simulink model "Feeder_1"  (Simulink 8.8)
settings: Solver=ode4  StartTime=0.0  StopTime=inf  FixedStep=Ts  RelTol=1e-3  EnableMultiTasking=on
PreLoadFcn:
  | Ts=125e-6;Core_Num = 0; np=1; nq=1; Vmin=.9;
PostLoadFcn:
  | Ts=125e-6;Core_Num = 0; np=1; nq=1; Vmin=.9;
InitFcn:
  | Ts=125e-6;Core_Num = 0; np=1; nq=1; Vmin=.9;
undefined symbols (not defined in the file or in its folder): another_event_name, DiscIntNeverNeededParam, I, j, Left, my_event_name, Right, type, V, X
libraries: powerlib x316, powerlib_meascontrol x227, simulink_extras x78, simulink x25, rtio_generic_c37_118 x22, ssn_lib x9, rtlab x6, powerlib_extras x3, artemis x1, rtio_opalrt_ml605ex1 x1, rtio_spectracom x1, rtio_generic_ethernet x1
(part 4 of 14)

== system Feeder_1/SM_NG/Single-Phase Dynamic Load36 ==
  PQ : Inport
  Controlled Current Source : powerlib/Electrical Sources/Controlled Current Source  Initialize=on  Source_Type=AC  Amplitude=0  Phase=0  Frequency=0  Measurements=None
  Ground52 : powerlib/Elements/Ground  LConnTagsString=a
  Voltage Measurement1 : powerlib/Measurements/Voltage Measurement  PhasorSimulation=off  OutputType=Complex  PSBequivalent=0
  model : Subsystem
  a : PMIOPort  Tag=PMCPort  Port=1  Side=Right
  wires:
  PQ/1 -> model/2(PQ)
  Voltage Measurement1/1 -> model/1(v)
  model/1(i) -> Controlled Current Source/1
  connections:
  Voltage Measurement1/LConn1 -- a/RConn1 -- Controlled Current Source/RConn1
  Voltage Measurement1/LConn2 -- Ground52/LConn1 -- Controlled Current Source/LConn1

== system Feeder_1/SM_NG/Single-Phase Dynamic Load37 ==
  PQ : Inport
  Controlled Current Source : powerlib/Electrical Sources/Controlled Current Source  Initialize=on  Source_Type=AC  Amplitude=0  Phase=0  Frequency=0  Measurements=None
  Ground52 : powerlib/Elements/Ground  LConnTagsString=a
  Voltage Measurement1 : powerlib/Measurements/Voltage Measurement  PhasorSimulation=off  OutputType=Complex  PSBequivalent=0
  model : Subsystem
  a : PMIOPort  Tag=PMCPort  Port=1  Side=Right
  wires:
  PQ/1 -> model/2(PQ)
  Voltage Measurement1/1 -> model/1(v)
  model/1(i) -> Controlled Current Source/1
  connections:
  Voltage Measurement1/LConn1 -- a/RConn1 -- Controlled Current Source/RConn1
  Ground52/LConn1 -- Voltage Measurement1/LConn2 -- Controlled Current Source/LConn1

== system Feeder_1/SM_NG/Single-Phase Dynamic Load38 ==
  PQ : Inport
  Controlled Current Source : powerlib/Electrical Sources/Controlled Current Source  Initialize=on  Source_Type=AC  Amplitude=0  Phase=0  Frequency=0  Measurements=None
  Ground52 : powerlib/Elements/Ground  LConnTagsString=a
  Voltage Measurement1 : powerlib/Measurements/Voltage Measurement  PhasorSimulation=off  OutputType=Complex  PSBequivalent=0
  model : Subsystem
  a : PMIOPort  Tag=PMCPort  Port=1  Side=Right
  wires:
  PQ/1 -> model/2(PQ)
  Voltage Measurement1/1 -> model/1(v)
  model/1(i) -> Controlled Current Source/1
  connections:
  Voltage Measurement1/LConn1 -- a/RConn1 -- Controlled Current Source/RConn1
  Voltage Measurement1/LConn2 -- Ground52/LConn1 -- Controlled Current Source/LConn1

== system Feeder_1/SM_NG/Single-Phase Dynamic Load39 ==
  PQ : Inport
  Controlled Current Source : powerlib/Electrical Sources/Controlled Current Source  Initialize=on  Source_Type=AC  Amplitude=0  Phase=0  Frequency=0  Measurements=None
  Ground52 : powerlib/Elements/Ground  LConnTagsString=a
  Voltage Measurement1 : powerlib/Measurements/Voltage Measurement  PhasorSimulation=off  OutputType=Complex  PSBequivalent=0
  model : Subsystem
  a : PMIOPort  Tag=PMCPort  Port=1  Side=Right
  wires:
  PQ/1 -> model/2(PQ)
  Voltage Measurement1/1 -> model/1(v)
  model/1(i) -> Controlled Current Source/1
  connections:
  Voltage Measurement1/LConn1 -- a/RConn1 -- Controlled Current Source/RConn1
  Voltage Measurement1/LConn2 -- Ground52/LConn1 -- Controlled Current Source/LConn1

== system Feeder_1/SM_NG/Single-Phase Dynamic Load40 ==
  PQ : Inport
  Controlled Current Source : powerlib/Electrical Sources/Controlled Current Source  Initialize=on  Source_Type=AC  Amplitude=0  Phase=0  Frequency=0  Measurements=None
  Ground57 : powerlib/Elements/Ground  LConnTagsString=a
  Voltage Measurement1 : powerlib/Measurements/Voltage Measurement  PhasorSimulation=off  OutputType=Complex  PSBequivalent=0
  model : Subsystem
  a : PMIOPort  Tag=PMCPort  Port=1  Side=Right
  wires:
  PQ/1 -> model/2(PQ)
  Voltage Measurement1/1 -> model/1(v)
  model/1(i) -> Controlled Current Source/1
  connections:
  Voltage Measurement1/LConn1 -- a/RConn1 -- Controlled Current Source/RConn1
  Voltage Measurement1/LConn2 -- Ground57/LConn1 -- Controlled Current Source/LConn1

== system Feeder_1/SM_NG/Single-Phase Dynamic Load41 ==
  PQ : Inport
  Controlled Current Source : powerlib/Electrical Sources/Controlled Current Source  Initialize=on  Source_Type=AC  Amplitude=0  Phase=0  Frequency=0  Measurements=None
  Ground57 : powerlib/Elements/Ground  LConnTagsString=a
  Voltage Measurement1 : powerlib/Measurements/Voltage Measurement  PhasorSimulation=off  OutputType=Complex  PSBequivalent=0
  model : Subsystem
  a : PMIOPort  Tag=PMCPort  Port=1  Side=Right
  wires:
  PQ/1 -> model/2(PQ)
  Voltage Measurement1/1 -> model/1(v)
  model/1(i) -> Controlled Current Source/1
  connections:
  Voltage Measurement1/LConn1 -- a/RConn1 -- Controlled Current Source/RConn1
  Voltage Measurement1/LConn2 -- Ground57/LConn1 -- Controlled Current Source/LConn1

== system Feeder_1/SM_NG/Single-Phase Dynamic Load42 ==
  PQ : Inport
  Controlled Current Source : powerlib/Electrical Sources/Controlled Current Source  Initialize=on  Source_Type=AC  Amplitude=0  Phase=0  Frequency=0  Measurements=None
  Ground50 : powerlib/Elements/Ground  LConnTagsString=a
  Voltage Measurement1 : powerlib/Measurements/Voltage Measurement  PhasorSimulation=off  OutputType=Complex  PSBequivalent=0
  model : Subsystem
  a : PMIOPort  Tag=PMCPort  Port=1  Side=Right
  wires:
  PQ/1 -> model/2(PQ)
  Voltage Measurement1/1 -> model/1(v)
  model/1(i) -> Controlled Current Source/1
  connections:
  Voltage Measurement1/LConn1 -- a/RConn1 -- Controlled Current Source/RConn1
  Voltage Measurement1/LConn2 -- Ground50/LConn1 -- Controlled Current Source/LConn1

== system Feeder_1/SM_NG/Single-Phase Dynamic Load43 ==
  PQ : Inport
  Controlled Current Source : powerlib/Electrical Sources/Controlled Current Source  Initialize=on  Source_Type=AC  Amplitude=0  Phase=0  Frequency=0  Measurements=None
  Ground57 : powerlib/Elements/Ground  LConnTagsString=a
  Voltage Measurement1 : powerlib/Measurements/Voltage Measurement  PhasorSimulation=off  OutputType=Complex  PSBequivalent=0
  model : Subsystem
  a : PMIOPort  Tag=PMCPort  Port=1  Side=Right
  wires:
  PQ/1 -> model/2(PQ)
  Voltage Measurement1/1 -> model/1(v)
  model/1(i) -> Controlled Current Source/1
  connections:
  Voltage Measurement1/LConn1 -- a/RConn1 -- Controlled Current Source/RConn1
  Voltage Measurement1/LConn2 -- Ground57/LConn1 -- Controlled Current Source/LConn1

== system Feeder_1/SM_NG/Single-Phase Dynamic Load44 ==
  PQ : Inport
  Controlled Current Source : powerlib/Electrical Sources/Controlled Current Source  Initialize=on  Source_Type=AC  Amplitude=0  Phase=0  Frequency=0  Measurements=None
  Ground57 : powerlib/Elements/Ground  LConnTagsString=a
  Voltage Measurement1 : powerlib/Measurements/Voltage Measurement  PhasorSimulation=off  OutputType=Complex  PSBequivalent=0
  model : Subsystem
  a : PMIOPort  Tag=PMCPort  Port=1  Side=Right
  wires:
  PQ/1 -> model/2(PQ)
  Voltage Measurement1/1 -> model/1(v)
  model/1(i) -> Controlled Current Source/1
  connections:
  Voltage Measurement1/LConn1 -- a/RConn1 -- Controlled Current Source/RConn1
  Voltage Measurement1/LConn2 -- Ground57/LConn1 -- Controlled Current Source/LConn1

== system Feeder_1/SM_NG/Single-Phase Dynamic Load45 ==
  PQ : Inport
  Controlled Current Source : powerlib/Electrical Sources/Controlled Current Source  Initialize=on  Source_Type=AC  Amplitude=0  Phase=0  Frequency=0  Measurements=None
  Ground57 : powerlib/Elements/Ground  LConnTagsString=a
  Voltage Measurement1 : powerlib/Measurements/Voltage Measurement  PhasorSimulation=off  OutputType=Complex  PSBequivalent=0
  model : Subsystem
  a : PMIOPort  Tag=PMCPort  Port=1  Side=Right
  wires:
  PQ/1 -> model/2(PQ)
  Voltage Measurement1/1 -> model/1(v)
  model/1(i) -> Controlled Current Source/1
  connections:
  Voltage Measurement1/LConn1 -- a/RConn1 -- Controlled Current Source/RConn1
  Voltage Measurement1/LConn2 -- Ground57/LConn1 -- Controlled Current Source/LConn1

== system Feeder_1/SM_NG/Single-Phase Dynamic Load46 ==
  PQ : Inport
  Controlled Current Source : powerlib/Electrical Sources/Controlled Current Source  Initialize=on  Source_Type=AC  Amplitude=0  Phase=0  Frequency=0  Measurements=None
  Ground57 : powerlib/Elements/Ground  LConnTagsString=a
  Voltage Measurement1 : powerlib/Measurements/Voltage Measurement  PhasorSimulation=off  OutputType=Complex  PSBequivalent=0
  model : Subsystem
  a : PMIOPort  Tag=PMCPort  Port=1  Side=Right
  wires:
  PQ/1 -> model/2(PQ)
  Voltage Measurement1/1 -> model/1(v)
  model/1(i) -> Controlled Current Source/1
  connections:
  Voltage Measurement1/LConn1 -- a/RConn1 -- Controlled Current Source/RConn1
  Voltage Measurement1/LConn2 -- Ground57/LConn1 -- Controlled Current Source/LConn1

== system Feeder_1/SM_NG/Single-Phase Dynamic Load47 ==
  PQ : Inport
  Controlled Current Source : powerlib/Electrical Sources/Controlled Current Source  Initialize=on  Source_Type=AC  Amplitude=0  Phase=0  Frequency=0  Measurements=None
  Ground52 : powerlib/Elements/Ground  LConnTagsString=a
  Voltage Measurement1 : powerlib/Measurements/Voltage Measurement  PhasorSimulation=off  OutputType=Complex  PSBequivalent=0
  model : Subsystem
  a : PMIOPort  Tag=PMCPort  Port=1  Side=Right
  wires:
  PQ/1 -> model/2(PQ)
  Voltage Measurement1/1 -> model/1(v)
  model/1(i) -> Controlled Current Source/1
  connections:
  Voltage Measurement1/LConn1 -- a/RConn1 -- Controlled Current Source/RConn1
  Voltage Measurement1/LConn2 -- Ground52/LConn1 -- Controlled Current Source/LConn1

== system Feeder_1/SM_NG/Single-Phase Dynamic Load48 ==
  PQ : Inport
  Controlled Current Source : powerlib/Electrical Sources/Controlled Current Source  Initialize=on  Source_Type=AC  Amplitude=0  Phase=0  Frequency=0  Measurements=None
  Ground52 : powerlib/Elements/Ground  LConnTagsString=a
  Voltage Measurement1 : powerlib/Measurements/Voltage Measurement  PhasorSimulation=off  OutputType=Complex  PSBequivalent=0
  model : Subsystem
  a : PMIOPort  Tag=PMCPort  Port=1  Side=Right
  wires:
  PQ/1 -> model/2(PQ)
  Voltage Measurement1/1 -> model/1(v)
  model/1(i) -> Controlled Current Source/1
  connections:
  Voltage Measurement1/LConn1 -- a/RConn1 -- Controlled Current Source/RConn1
  Voltage Measurement1/LConn2 -- Ground52/LConn1 -- Controlled Current Source/LConn1

== system Feeder_1/SM_NG/Single-Phase Dynamic Load49 ==
  PQ : Inport
  Controlled Current Source : powerlib/Electrical Sources/Controlled Current Source  Initialize=on  Source_Type=AC  Amplitude=0  Phase=0  Frequency=0  Measurements=None
  Ground52 : powerlib/Elements/Ground  LConnTagsString=a
  Voltage Measurement1 : powerlib/Measurements/Voltage Measurement  PhasorSimulation=off  OutputType=Complex  PSBequivalent=0
  model : Subsystem
  a : PMIOPort  Tag=PMCPort  Port=1  Side=Right
  wires:
  PQ/1 -> model/2(PQ)
  Voltage Measurement1/1 -> model/1(v)
  model/1(i) -> Controlled Current Source/1
  connections:
  Voltage Measurement1/LConn1 -- a/RConn1 -- Controlled Current Source/RConn1
  Voltage Measurement1/LConn2 -- Ground52/LConn1 -- Controlled Current Source/LConn1

== system Feeder_1/SM_NG/Single-Phase Dynamic Load50 ==
  PQ : Inport
  Controlled Current Source : powerlib/Electrical Sources/Controlled Current Source  Initialize=on  Source_Type=AC  Amplitude=0  Phase=0  Frequency=0  Measurements=None
  Ground59 : powerlib/Elements/Ground  LConnTagsString=a
  Voltage Measurement1 : powerlib/Measurements/Voltage Measurement  PhasorSimulation=off  OutputType=Complex  PSBequivalent=0
  model : Subsystem
  a : PMIOPort  Tag=PMCPort  Port=1  Side=Right
  wires:
  PQ/1 -> model/2(PQ)
  Voltage Measurement1/1 -> model/1(v)
  model/1(i) -> Controlled Current Source/1
  connections:
  Voltage Measurement1/LConn1 -- a/RConn1 -- Controlled Current Source/RConn1
  Voltage Measurement1/LConn2 -- Ground59/LConn1 -- Controlled Current Source/LConn1

== system Feeder_1/SM_NG/Single-Phase Dynamic Load51 ==
  PQ : Inport
  Controlled Current Source : powerlib/Electrical Sources/Controlled Current Source  Initialize=on  Source_Type=AC  Amplitude=0  Phase=0  Frequency=0  Measurements=None
  Ground59 : powerlib/Elements/Ground  LConnTagsString=a
  Voltage Measurement1 : powerlib/Measurements/Voltage Measurement  PhasorSimulation=off  OutputType=Complex  PSBequivalent=0
  model : Subsystem
  a : PMIOPort  Tag=PMCPort  Port=1  Side=Right
  wires:
  PQ/1 -> model/2(PQ)
  Voltage Measurement1/1 -> model/1(v)
  model/1(i) -> Controlled Current Source/1
  connections:
  Voltage Measurement1/LConn1 -- a/RConn1 -- Controlled Current Source/RConn1
  Voltage Measurement1/LConn2 -- Ground59/LConn1 -- Controlled Current Source/LConn1

== system Feeder_1/SM_NG/Single-Phase Dynamic Load52 ==
  PQ : Inport
  Controlled Current Source : powerlib/Electrical Sources/Controlled Current Source  Initialize=on  Source_Type=AC  Amplitude=0  Phase=0  Frequency=0  Measurements=None
  Ground59 : powerlib/Elements/Ground  LConnTagsString=a
  Voltage Measurement1 : powerlib/Measurements/Voltage Measurement  PhasorSimulation=off  OutputType=Complex  PSBequivalent=0
  model : Subsystem
  a : PMIOPort  Tag=PMCPort  Port=1  Side=Right
  wires:
  PQ/1 -> model/2(PQ)
  Voltage Measurement1/1 -> model/1(v)
  model/1(i) -> Controlled Current Source/1
  connections:
  Voltage Measurement1/LConn1 -- a/RConn1 -- Controlled Current Source/RConn1
  Voltage Measurement1/LConn2 -- Controlled Current Source/LConn1 -- Ground59/LConn1

== system Feeder_1/SM_NG/Single-Phase Dynamic Load53 ==
  PQ : Inport
  Controlled Current Source : powerlib/Electrical Sources/Controlled Current Source  Initialize=on  Source_Type=AC  Amplitude=0  Phase=0  Frequency=0  Measurements=None
  Ground62 : powerlib/Elements/Ground  LConnTagsString=a
  Voltage Measurement1 : powerlib/Measurements/Voltage Measurement  PhasorSimulation=off  OutputType=Complex  PSBequivalent=0
  model : Subsystem
  a : PMIOPort  Tag=PMCPort  Port=1  Side=Right
  wires:
  PQ/1 -> model/2(PQ)
  Voltage Measurement1/1 -> model/1(v)
  model/1(i) -> Controlled Current Source/1
  connections:
  Voltage Measurement1/LConn1 -- a/RConn1 -- Controlled Current Source/RConn1
  Voltage Measurement1/LConn2 -- Ground62/LConn1 -- Controlled Current Source/LConn1

== system Feeder_1/SM_NG/Single-Phase Dynamic Load54 ==
  PQ : Inport
  Controlled Current Source : powerlib/Electrical Sources/Controlled Current Source  Initialize=on  Source_Type=AC  Amplitude=0  Phase=0  Frequency=0  Measurements=None
  Ground64 : powerlib/Elements/Ground  LConnTagsString=a
  Voltage Measurement1 : powerlib/Measurements/Voltage Measurement  PhasorSimulation=off  OutputType=Complex  PSBequivalent=0
  model : Subsystem
  a : PMIOPort  Tag=PMCPort  Port=1  Side=Right
  wires:
  PQ/1 -> model/2(PQ)
  Voltage Measurement1/1 -> model/1(v)
  model/1(i) -> Controlled Current Source/1
  connections:
  Voltage Measurement1/LConn1 -- a/RConn1 -- Controlled Current Source/RConn1
  Voltage Measurement1/LConn2 -- Ground64/LConn1 -- Controlled Current Source/LConn1

== system Feeder_1/SM_NG/Single-Phase Dynamic Load55 ==
  PQ : Inport
  Controlled Current Source : powerlib/Electrical Sources/Controlled Current Source  Initialize=on  Source_Type=AC  Amplitude=0  Phase=0  Frequency=0  Measurements=None
  Ground62 : powerlib/Elements/Ground  LConnTagsString=a
  Voltage Measurement1 : powerlib/Measurements/Voltage Measurement  PhasorSimulation=off  OutputType=Complex  PSBequivalent=0
  model : Subsystem
  a : PMIOPort  Tag=PMCPort  Port=1  Side=Right
  wires:
  PQ/1 -> model/2(PQ)
  Voltage Measurement1/1 -> model/1(v)
  model/1(i) -> Controlled Current Source/1
  connections:
  Voltage Measurement1/LConn1 -- a/RConn1 -- Controlled Current Source/RConn1
  Voltage Measurement1/LConn2 -- Ground62/LConn1 -- Controlled Current Source/LConn1

== system Feeder_1/SM_NG/Single-Phase Dynamic Load56 ==
  PQ : Inport
  Controlled Current Source : powerlib/Electrical Sources/Controlled Current Source  Initialize=on  Source_Type=AC  Amplitude=0  Phase=0  Frequency=0  Measurements=None
  Ground50 : powerlib/Elements/Ground  LConnTagsString=a
  Voltage Measurement1 : powerlib/Measurements/Voltage Measurement  PhasorSimulation=off  OutputType=Complex  PSBequivalent=0
  model : Subsystem
  a : PMIOPort  Tag=PMCPort  Port=1  Side=Right
  wires:
  PQ/1 -> model/2(PQ)
  Voltage Measurement1/1 -> model/1(v)
  model/1(i) -> Controlled Current Source/1
  connections:
  Voltage Measurement1/LConn1 -- a/RConn1 -- Controlled Current Source/RConn1
  Voltage Measurement1/LConn2 -- Ground50/LConn1 -- Controlled Current Source/LConn1

== system Feeder_1/SM_NG/Single-Phase Dynamic Load57 ==
  PQ : Inport
  Controlled Current Source : powerlib/Electrical Sources/Controlled Current Source  Initialize=on  Source_Type=AC  Amplitude=0  Phase=0  Frequency=0  Measurements=None
  Ground51 : powerlib/Elements/Ground  LConnTagsString=a
  Voltage Measurement1 : powerlib/Measurements/Voltage Measurement  PhasorSimulation=off  OutputType=Complex  PSBequivalent=0
  model : Subsystem
  a : PMIOPort  Tag=PMCPort  Port=1  Side=Right
  wires:
  PQ/1 -> model/2(PQ)
  Voltage Measurement1/1 -> model/1(v)
  model/1(i) -> Controlled Current Source/1
  connections:
  Voltage Measurement1/LConn1 -- a/RConn1 -- Controlled Current Source/RConn1
  Voltage Measurement1/LConn2 -- Ground51/LConn1 -- Controlled Current Source/LConn1

== system Feeder_1/SM_NG/Single-Phase Dynamic Load58 ==
  PQ : Inport
  Controlled Current Source : powerlib/Electrical Sources/Controlled Current Source  Initialize=on  Source_Type=AC  Amplitude=0  Phase=0  Frequency=0  Measurements=None
  Ground51 : powerlib/Elements/Ground  LConnTagsString=a
  Voltage Measurement1 : powerlib/Measurements/Voltage Measurement  PhasorSimulation=off  OutputType=Complex  PSBequivalent=0
  model : Subsystem
  a : PMIOPort  Tag=PMCPort  Port=1  Side=Right
  wires:
  PQ/1 -> model/2(PQ)
  Voltage Measurement1/1 -> model/1(v)
  model/1(i) -> Controlled Current Source/1
  connections:
  Voltage Measurement1/LConn1 -- a/RConn1 -- Controlled Current Source/RConn1
  Voltage Measurement1/LConn2 -- Ground51/LConn1 -- Controlled Current Source/LConn1

== system Feeder_1/SM_NG/Single-Phase Dynamic Load59 ==
  PQ : Inport
  Controlled Current Source : powerlib/Electrical Sources/Controlled Current Source  Initialize=on  Source_Type=AC  Amplitude=0  Phase=0  Frequency=0  Measurements=None
  Ground51 : powerlib/Elements/Ground  LConnTagsString=a
  Voltage Measurement1 : powerlib/Measurements/Voltage Measurement  PhasorSimulation=off  OutputType=Complex  PSBequivalent=0
  model : Subsystem
  a : PMIOPort  Tag=PMCPort  Port=1  Side=Right
  wires:
  PQ/1 -> model/2(PQ)
  Voltage Measurement1/1 -> model/1(v)
  model/1(i) -> Controlled Current Source/1
  connections:
  Voltage Measurement1/LConn1 -- a/RConn1 -- Controlled Current Source/RConn1
  Voltage Measurement1/LConn2 -- Controlled Current Source/LConn1 -- Ground51/LConn1

== system Feeder_1/SM_NG/Single-Phase Dynamic Load60 ==
  PQ : Inport
  Controlled Current Source : powerlib/Electrical Sources/Controlled Current Source  Initialize=on  Source_Type=AC  Amplitude=0  Phase=0  Frequency=0  Measurements=None
  Ground52 : powerlib/Elements/Ground  LConnTagsString=a
  Voltage Measurement1 : powerlib/Measurements/Voltage Measurement  PhasorSimulation=off  OutputType=Complex  PSBequivalent=0
  model : Subsystem
  a : PMIOPort  Tag=PMCPort  Port=1  Side=Right
  wires:
  PQ/1 -> model/2(PQ)
  Voltage Measurement1/1 -> model/1(v)
  model/1(i) -> Controlled Current Source/1
  connections:
  Voltage Measurement1/LConn1 -- a/RConn1 -- Controlled Current Source/RConn1
  Voltage Measurement1/LConn2 -- Ground52/LConn1 -- Controlled Current Source/LConn1

== system Feeder_1/SM_NG/Subsystem ==
  Single-Phase Voltage Regulator1 : Subsystem  mask(Single-Phase Voltage Regulator){pNom=3330e3, fNom=60, vNom=13.8e3/sqrt(3), rFdrCurrent=3330e3/(13.8e3*sqrt(3)), iTapNo=0, vRef=122.4/120, bandwidth=1.25, totalDelay=30, rComp=6, xComp=6}
      mask prompts: pNom "Nominal power (VA)"; fNom "Nominal frequency (Hz)"; vNom "Nominal voltage (Vrms)"; rFdrCurrent "Rated feeder current (A)"; iTapNo "Initial tap number (-17 < x < 17)"; vRef "Reference voltage (P.U.)"; bandwidth "Bandwidth (P.U.)"; totalDelay "Time delay (s) + mechanical delay (s)"; rComp "R (V)"; xComp "X (V)"
      mask help:
      | The single-phase VR is designed for MV and primary LV systems. It consists of a 16-tap autotransformer and a step voltage regulating relay.
      |
      | The VR contains a reversing switch enabling a +/- 10% regulating range, in 16 steps up and 16 steps down.
      |
      | The VR performs a tap change if:
      |     abs(V-Vref) > Bandwidth/2  during a time  t > total delay.
      |
      | Note that R and X, specified on the "Compensator Settings" tab, are needed to dial on the control box of the regulator and are in units of volts.
      |
      | More info on VR modeling:
      |     W. H. Kersting, ribution Feeder Voltage Regulation Control,6, March/April 2010.
      mask init:
      | ptRatio = vNom / 120;  % Compensator and logic circuits are rated for 120V. 
      | ctRatio = rFdrCurrent / 0.2;  % The rated secondary current is 0.2A.
      | 
      | % Since the rated secondary current of the CT is 0.2A, the impedance of the
      | % analog compensator is obtained from the following equations to result in
      | % the voltage drop specified by Zcomp.
      | r = rComp / 0.2;   
      | x = xComp / 0.2;
      mask Display: image(imread('VR.jpg'))
  Single-Phase Voltage Regulator2 : Subsystem  mask(Single-Phase Voltage Regulator){pNom=3330e3, fNom=60, vNom=13.8e3/sqrt(3), rFdrCurrent=3330e3/(13.8e3*sqrt(3)), iTapNo=-2, vRef=122.4/120, bandwidth=1.25, totalDelay=30, rComp=6, xComp=6}
      mask prompts: pNom "Nominal power (VA)"; fNom "Nominal frequency (Hz)"; vNom "Nominal voltage (Vrms)"; rFdrCurrent "Rated feeder current (A)"; iTapNo "Initial tap number (-17 < x < 17)"; vRef "Reference voltage (P.U.)"; bandwidth "Bandwidth (P.U.)"; totalDelay "Time delay (s) + mechanical delay (s)"; rComp "R (V)"; xComp "X (V)"
      mask help:
      | The single-phase VR is designed for MV and primary LV systems. It consists of a 16-tap autotransformer and a step voltage regulating relay.
      |
      | The VR contains a reversing switch enabling a +/- 10% regulating range, in 16 steps up and 16 steps down.
      |
      | The VR performs a tap change if:
      |     abs(V-Vref) > Bandwidth/2  during a time  t > total delay.
      |
      | Note that R and X, specified on the "Compensator Settings" tab, are needed to dial on the control box of the regulator and are in units of volts.
      |
      | More info on VR modeling:
      |     W. H. Kersting, ribution Feeder Voltage Regulation Control,6, March/April 2010.
      mask init: same as Feeder_1/SM_NG/Subsystem/Single-Phase Voltage Regulator1
      mask Display: image(imread('VR.jpg'))
  Single-Phase Voltage Regulator3 : Subsystem  mask(Single-Phase Voltage Regulator){pNom=3330e3, fNom=60, vNom=13.8e3/sqrt(3), rFdrCurrent=3330e3/(13.8e3*sqrt(3)), iTapNo=0, vRef=122.4/120, bandwidth=1.25, totalDelay=30, rComp=6, xComp=6}
      mask prompts: pNom "Nominal power (VA)"; fNom "Nominal frequency (Hz)"; vNom "Nominal voltage (Vrms)"; rFdrCurrent "Rated feeder current (A)"; iTapNo "Initial tap number (-17 < x < 17)"; vRef "Reference voltage (P.U.)"; bandwidth "Bandwidth (P.U.)"; totalDelay "Time delay (s) + mechanical delay (s)"; rComp "R (V)"; xComp "X (V)"
      mask help:
      | The single-phase VR is designed for MV and primary LV systems. It consists of a 16-tap autotransformer and a step voltage regulating relay.
      |
      | The VR contains a reversing switch enabling a +/- 10% regulating range, in 16 steps up and 16 steps down.
      |
      | The VR performs a tap change if:
      |     abs(V-Vref) > Bandwidth/2  during a time  t > total delay.
      |
      | Note that R and X, specified on the "Compensator Settings" tab, are needed to dial on the control box of the regulator and are in units of volts.
      |
      | More info on VR modeling:
      |     W. H. Kersting, ribution Feeder Voltage Regulation Control,6, March/April 2010.
      mask init: same as Feeder_1/SM_NG/Subsystem/Single-Phase Voltage Regulator1
      mask Display: image(imread('VR.jpg'))
  Conn1 : PMIOPort  Port=1  Side=Left
  Conn2 : PMIOPort  Port=2  Side=Right
  Conn3 : PMIOPort  Port=3  Side=Left
  Conn4 : PMIOPort  Port=4  Side=Right
  Conn5 : PMIOPort  Port=5  Side=Left
  Conn6 : PMIOPort  Port=6  Side=Right
  Out1 : Outport
  Out2 : Outport  Port=2
  Out3 : Outport  Port=3
  wires:
  Single-Phase Voltage Regulator3/1(tapNo) -> Out1/1
  Single-Phase Voltage Regulator1/1(tapNo) -> Out3/1
  Single-Phase Voltage Regulator2/1(tapNo) -> Out2/1
  connections:
  Conn4/RConn1 -- Single-Phase Voltage Regulator2/RConn1
  Conn6/RConn1 -- Single-Phase Voltage Regulator1/RConn1
  Conn2/RConn1 -- Single-Phase Voltage Regulator3/RConn1
  Single-Phase Voltage Regulator1/LConn1 -- Conn5/RConn1
  Single-Phase Voltage Regulator2/LConn1 -- Conn3/RConn1
  Single-Phase Voltage Regulator3/LConn1 -- Conn1/RConn1

== system Feeder_1/SM_NG/Timestamp selector ==
  ts_in : Inport
  Constant5 : Constant  Value=1000
  Demux : Demux  Outputs=7
  Mux : Mux  Inputs=3
  Terminator{,1..3} (4 alike) : Terminator
  nS to uS : Product  Inputs=*/
  ts_out : Outport
  wires:
  Demux/1 -> Terminator/1
  Demux/2 -> Terminator1/1
  Demux/3 -> Terminator2/1
  Demux/4 -> Terminator3/1
  Demux/5 -> [ns]
  Demux/6 -> [epoch]
  ts_in/1 -> Demux/1
  [epoch] -> Mux/2
  Demux/7 -> [sync]
  [sync] -> Mux/1
  Mux/1 -> ts_out/1
  Constant5/1 -> nS to uS/2
  [ns] -> nS to uS/1
  nS to uS/1 -> Mux/3

== system Feeder_1/SS_PMU/Subsystem1 ==
  Measurements : Inport
  Demux7 : Demux  Outputs=6
  Demux8 : Demux  Outputs=6
  Mux5 : Mux  Inputs=12
  Subsystem : Subsystem
  Phasors : Outport
  Phasor_Freq : Outport  Port=2
  FROC : Outport  Port=3
  wires:
  Mux5/1 -> Phasors/1
  Demux7/4 -> [Phase_Va]
  Demux7/1 -> [Mag_Va]
  Demux7/2 -> [Mag_Vb]
  Demux7/3 -> [Mag_Vc]
  Subsystem/1(Phasors_Vabc) -> Demux7/1
  Demux7/6 -> [Phase_Vc]
  Demux7/5 -> [Phase_Vb]
  Subsystem/3(Phasor_Freq) -> Phasor_Freq/1
  Measurements/1 -> Subsystem/1(Measurements1)
  Subsystem/4(Phasor_DTFreq) -> FROC/1
  Demux8/2 -> [Mag_Ib]
  Demux8/4 -> [Phase_Ia]
  Demux8/5 -> [Phase_Ib]
  Subsystem/2(Phasors_Iabc) -> Demux8/1
  Demux8/3 -> [Mag_Ic]
  Demux8/1 -> [Mag_Ia]
  Demux8/6 -> [Phase_Ic]
  [Phase_Ic] -> Mux5/12
  [Mag_Ic] -> Mux5/11
  [Phase_Ib] -> Mux5/10
  [Mag_Ib] -> Mux5/9
  [Phase_Ia] -> Mux5/8
  [Mag_Ia] -> Mux5/7
  [Phase_Vc] -> Mux5/6
  [Mag_Vc] -> Mux5/5
  [Phase_Vb] -> Mux5/4
  [Mag_Vb] -> Mux5/3
  [Phase_Va] -> Mux5/2
  [Mag_Va] -> Mux5/1

== system Feeder_1/SS_PMU/Subsystem10 ==
  Measurements : Inport
  Demux7 : Demux  Outputs=6
  Demux8 : Demux  Outputs=6
  Mux5 : Mux  Inputs=12
  Subsystem : Subsystem
  Phasors : Outport
  Phasor_Freq : Outport  Port=2
  FROC : Outport  Port=3
  wires:
  Mux5/1 -> Phasors/1
  Demux7/4 -> [Phase_Va]
  Demux7/1 -> [Mag_Va]
  Demux7/2 -> [Mag_Vb]
  Demux7/3 -> [Mag_Vc]
  Subsystem/1(Phasors_Vabc) -> Demux7/1
  Demux7/6 -> [Phase_Vc]
  Demux7/5 -> [Phase_Vb]
  Subsystem/3(Phasor_Freq) -> Phasor_Freq/1
  Measurements/1 -> Subsystem/1(Measurements1)
  Subsystem/4(Phasor_DTFreq) -> FROC/1
  Demux8/2 -> [Mag_Ib]
  Demux8/4 -> [Phase_Ia]
  Demux8/5 -> [Phase_Ib]
  Subsystem/2(Phasors_Iabc) -> Demux8/1
  Demux8/3 -> [Mag_Ic]
  Demux8/1 -> [Mag_Ia]
  Demux8/6 -> [Phase_Ic]
  [Phase_Ic] -> Mux5/12
  [Mag_Ic] -> Mux5/11
  [Phase_Ib] -> Mux5/10
  [Mag_Ib] -> Mux5/9
  [Phase_Ia] -> Mux5/8
  [Mag_Ia] -> Mux5/7
  [Phase_Vc] -> Mux5/6
  [Mag_Vc] -> Mux5/5
  [Phase_Vb] -> Mux5/4
  [Mag_Vb] -> Mux5/3
  [Phase_Va] -> Mux5/2
  [Mag_Va] -> Mux5/1

== system Feeder_1/SS_PMU/Subsystem11 ==
  Measurements : Inport
  Demux7 : Demux  Outputs=6
  Demux8 : Demux  Outputs=6
  Mux5 : Mux  Inputs=12
  Subsystem : Subsystem
  Phasors : Outport
  Phasor_Freq : Outport  Port=2
  FROC : Outport  Port=3
  wires:
  Mux5/1 -> Phasors/1
  Demux7/4 -> [Phase_Va]
  Demux7/1 -> [Mag_Va]
  Demux7/2 -> [Mag_Vb]
  Demux7/3 -> [Mag_Vc]
  Subsystem/1(Phasors_Vabc) -> Demux7/1
  Demux7/6 -> [Phase_Vc]
  Demux7/5 -> [Phase_Vb]
  Subsystem/3(Phasor_Freq) -> Phasor_Freq/1
  Measurements/1 -> Subsystem/1(Measurements1)
  Subsystem/4(Phasor_DTFreq) -> FROC/1
  Demux8/2 -> [Mag_Ib]
  Demux8/4 -> [Phase_Ia]
  Demux8/5 -> [Phase_Ib]
  Subsystem/2(Phasors_Iabc) -> Demux8/1
  Demux8/3 -> [Mag_Ic]
  Demux8/1 -> [Mag_Ia]
  Demux8/6 -> [Phase_Ic]
  [Phase_Ic] -> Mux5/12
  [Mag_Ic] -> Mux5/11
  [Phase_Ib] -> Mux5/10
  [Mag_Ib] -> Mux5/9
  [Phase_Ia] -> Mux5/8
  [Mag_Ia] -> Mux5/7
  [Phase_Vc] -> Mux5/6
  [Mag_Vc] -> Mux5/5
  [Phase_Vb] -> Mux5/4
  [Mag_Vb] -> Mux5/3
  [Phase_Va] -> Mux5/2
  [Mag_Va] -> Mux5/1

== system Feeder_1/SS_PMU/Subsystem12 ==
  Measurements : Inport
  Demux7 : Demux  Outputs=6
  Demux8 : Demux  Outputs=6
  Mux5 : Mux  Inputs=12
  Subsystem : Subsystem
  Phasors : Outport
  Phasor_Freq : Outport  Port=2
  FROC : Outport  Port=3
  wires:
  Mux5/1 -> Phasors/1
  Demux7/4 -> [Phase_Va]
  Demux7/1 -> [Mag_Va]
  Demux7/2 -> [Mag_Vb]
  Demux7/3 -> [Mag_Vc]
  Subsystem/1(Phasors_Vabc) -> Demux7/1
  Demux7/6 -> [Phase_Vc]
  Demux7/5 -> [Phase_Vb]
  Subsystem/3(Phasor_Freq) -> Phasor_Freq/1
  Measurements/1 -> Subsystem/1(Measurements1)
  Subsystem/4(Phasor_DTFreq) -> FROC/1
  Demux8/2 -> [Mag_Ib]
  Demux8/4 -> [Phase_Ia]
  Demux8/5 -> [Phase_Ib]
  Subsystem/2(Phasors_Iabc) -> Demux8/1
  Demux8/3 -> [Mag_Ic]
  Demux8/1 -> [Mag_Ia]
  Demux8/6 -> [Phase_Ic]
  [Phase_Ic] -> Mux5/12
  [Mag_Ic] -> Mux5/11
  [Phase_Ib] -> Mux5/10
  [Mag_Ib] -> Mux5/9
  [Phase_Ia] -> Mux5/8
  [Mag_Ia] -> Mux5/7
  [Phase_Vc] -> Mux5/6
  [Mag_Vc] -> Mux5/5
  [Phase_Vb] -> Mux5/4
  [Mag_Vb] -> Mux5/3
  [Phase_Va] -> Mux5/2
  [Mag_Va] -> Mux5/1

== system Feeder_1/SS_PMU/Subsystem13 ==
  Measurements : Inport
  Demux7 : Demux  Outputs=6
  Demux8 : Demux  Outputs=6
  Mux5 : Mux  Inputs=12
  Subsystem : Subsystem
  Phasors : Outport
  Phasor_Freq : Outport  Port=2
  FROC : Outport  Port=3
  wires:
  Mux5/1 -> Phasors/1
  Demux7/4 -> [Phase_Va]
  Demux7/1 -> [Mag_Va]
  Demux7/2 -> [Mag_Vb]
  Demux7/3 -> [Mag_Vc]
  Subsystem/1(Phasors_Vabc) -> Demux7/1
  Demux7/6 -> [Phase_Vc]
  Demux7/5 -> [Phase_Vb]
  Subsystem/3(Phasor_Freq) -> Phasor_Freq/1
  Measurements/1 -> Subsystem/1(Measurements1)
  Subsystem/4(Phasor_DTFreq) -> FROC/1
  Demux8/2 -> [Mag_Ib]
  Demux8/4 -> [Phase_Ia]
  Demux8/5 -> [Phase_Ib]
  Subsystem/2(Phasors_Iabc) -> Demux8/1
  Demux8/3 -> [Mag_Ic]
  Demux8/1 -> [Mag_Ia]
  Demux8/6 -> [Phase_Ic]
  [Phase_Ic] -> Mux5/12
  [Mag_Ic] -> Mux5/11
  [Phase_Ib] -> Mux5/10
  [Mag_Ib] -> Mux5/9
  [Phase_Ia] -> Mux5/8
  [Mag_Ia] -> Mux5/7
  [Phase_Vc] -> Mux5/6
  [Mag_Vc] -> Mux5/5
  [Phase_Vb] -> Mux5/4
  [Mag_Vb] -> Mux5/3
  [Phase_Va] -> Mux5/2
  [Mag_Va] -> Mux5/1

== system Feeder_1/SS_PMU/Subsystem14 ==
  Measurements : Inport
  Demux7 : Demux  Outputs=6
  Demux8 : Demux  Outputs=6
  Mux5 : Mux  Inputs=12
  Subsystem : Subsystem
  Phasors : Outport
  Phasor_Freq : Outport  Port=2
  FROC : Outport  Port=3
  wires:
  Mux5/1 -> Phasors/1
  Demux7/4 -> [Phase_Va]
  Demux7/1 -> [Mag_Va]
  Demux7/2 -> [Mag_Vb]
  Demux7/3 -> [Mag_Vc]
  Subsystem/1(Phasors_Vabc) -> Demux7/1
  Demux7/6 -> [Phase_Vc]
  Demux7/5 -> [Phase_Vb]
  Subsystem/3(Phasor_Freq) -> Phasor_Freq/1
  Measurements/1 -> Subsystem/1(Measurements1)
  Subsystem/4(Phasor_DTFreq) -> FROC/1
  Demux8/2 -> [Mag_Ib]
  Demux8/4 -> [Phase_Ia]
  Demux8/5 -> [Phase_Ib]
  Subsystem/2(Phasors_Iabc) -> Demux8/1
  Demux8/3 -> [Mag_Ic]
  Demux8/1 -> [Mag_Ia]
  Demux8/6 -> [Phase_Ic]
  [Phase_Ic] -> Mux5/12
  [Mag_Ic] -> Mux5/11
  [Phase_Ib] -> Mux5/10
  [Mag_Ib] -> Mux5/9
  [Phase_Ia] -> Mux5/8
  [Mag_Ia] -> Mux5/7
  [Phase_Vc] -> Mux5/6
  [Mag_Vc] -> Mux5/5
  [Phase_Vb] -> Mux5/4
  [Mag_Vb] -> Mux5/3
  [Phase_Va] -> Mux5/2
  [Mag_Va] -> Mux5/1

== system Feeder_1/SS_PMU/Subsystem15 ==
  Measurements : Inport
  Demux7 : Demux  Outputs=6
  Demux8 : Demux  Outputs=6
  Mux5 : Mux  Inputs=12
  Subsystem : Subsystem
  Phasors : Outport
  Phasor_Freq : Outport  Port=2
  FROC : Outport  Port=3
  wires:
  Mux5/1 -> Phasors/1
  Demux7/4 -> [Phase_Va]
  Demux7/1 -> [Mag_Va]
  Demux7/2 -> [Mag_Vb]
  Demux7/3 -> [Mag_Vc]
  Subsystem/1(Phasors_Vabc) -> Demux7/1
  Demux7/6 -> [Phase_Vc]
  Demux7/5 -> [Phase_Vb]
  Subsystem/3(Phasor_Freq) -> Phasor_Freq/1
  Measurements/1 -> Subsystem/1(Measurements1)
  Subsystem/4(Phasor_DTFreq) -> FROC/1
  Demux8/2 -> [Mag_Ib]
  Demux8/4 -> [Phase_Ia]
  Demux8/5 -> [Phase_Ib]
  Subsystem/2(Phasors_Iabc) -> Demux8/1
  Demux8/3 -> [Mag_Ic]
  Demux8/1 -> [Mag_Ia]
  Demux8/6 -> [Phase_Ic]
  [Phase_Ic] -> Mux5/12
  [Mag_Ic] -> Mux5/11
  [Phase_Ib] -> Mux5/10
  [Mag_Ib] -> Mux5/9
  [Phase_Ia] -> Mux5/8
  [Mag_Ia] -> Mux5/7
  [Phase_Vc] -> Mux5/6
  [Mag_Vc] -> Mux5/5
  [Phase_Vb] -> Mux5/4
  [Mag_Vb] -> Mux5/3
  [Phase_Va] -> Mux5/2
  [Mag_Va] -> Mux5/1

== system Feeder_1/SS_PMU/Subsystem16 ==
  Measurements : Inport
  Demux7 : Demux  Outputs=6
  Demux8 : Demux  Outputs=6
  Mux5 : Mux  Inputs=12
  Subsystem : Subsystem
  Phasors : Outport
  Phasor_Freq : Outport  Port=2
  FROC : Outport  Port=3
  wires:
  Mux5/1 -> Phasors/1
  Demux7/4 -> [Phase_Va]
  Demux7/1 -> [Mag_Va]
  Demux7/2 -> [Mag_Vb]
  Demux7/3 -> [Mag_Vc]
  Subsystem/1(Phasors_Vabc) -> Demux7/1
  Demux7/6 -> [Phase_Vc]
  Demux7/5 -> [Phase_Vb]
  Subsystem/3(Phasor_Freq) -> Phasor_Freq/1
  Measurements/1 -> Subsystem/1(Measurements1)
  Subsystem/4(Phasor_DTFreq) -> FROC/1
  Demux8/2 -> [Mag_Ib]
  Demux8/4 -> [Phase_Ia]
  Demux8/5 -> [Phase_Ib]
  Subsystem/2(Phasors_Iabc) -> Demux8/1
  Demux8/3 -> [Mag_Ic]
  Demux8/1 -> [Mag_Ia]
  Demux8/6 -> [Phase_Ic]
  [Phase_Ic] -> Mux5/12
  [Mag_Ic] -> Mux5/11
  [Phase_Ib] -> Mux5/10
  [Mag_Ib] -> Mux5/9
  [Phase_Ia] -> Mux5/8
  [Mag_Ia] -> Mux5/7
  [Phase_Vc] -> Mux5/6
  [Mag_Vc] -> Mux5/5
  [Phase_Vb] -> Mux5/4
  [Mag_Vb] -> Mux5/3
  [Phase_Va] -> Mux5/2
  [Mag_Va] -> Mux5/1

== system Feeder_1/SS_PMU/Subsystem17 ==
  Measurements : Inport
  Demux7 : Demux  Outputs=6
  Demux8 : Demux  Outputs=6
  Mux5 : Mux  Inputs=12
  Subsystem : Subsystem
  Phasors : Outport
  Phasor_Freq : Outport  Port=2
  FROC : Outport  Port=3
  wires:
  Mux5/1 -> Phasors/1
  Demux7/4 -> [Phase_Va]
  Demux7/1 -> [Mag_Va]
  Demux7/2 -> [Mag_Vb]
  Demux7/3 -> [Mag_Vc]
  Subsystem/1(Phasors_Vabc) -> Demux7/1
  Demux7/6 -> [Phase_Vc]
  Demux7/5 -> [Phase_Vb]
  Subsystem/3(Phasor_Freq) -> Phasor_Freq/1
  Measurements/1 -> Subsystem/1(Measurements1)
  Subsystem/4(Phasor_DTFreq) -> FROC/1
  Demux8/2 -> [Mag_Ib]
  Demux8/4 -> [Phase_Ia]
  Demux8/5 -> [Phase_Ib]
  Subsystem/2(Phasors_Iabc) -> Demux8/1
  Demux8/3 -> [Mag_Ic]
  Demux8/1 -> [Mag_Ia]
  Demux8/6 -> [Phase_Ic]
  [Phase_Ic] -> Mux5/12
  [Mag_Ic] -> Mux5/11
  [Phase_Ib] -> Mux5/10
  [Mag_Ib] -> Mux5/9
  [Phase_Ia] -> Mux5/8
  [Mag_Ia] -> Mux5/7
  [Phase_Vc] -> Mux5/6
  [Mag_Vc] -> Mux5/5
  [Phase_Vb] -> Mux5/4
  [Mag_Vb] -> Mux5/3
  [Phase_Va] -> Mux5/2
  [Mag_Va] -> Mux5/1

== system Feeder_1/SS_PMU/Subsystem18 ==
  Measurements : Inport
  Demux7 : Demux  Outputs=6
  Demux8 : Demux  Outputs=6
  Mux5 : Mux  Inputs=12
  Subsystem : Subsystem
  Phasors : Outport
  Phasor_Freq : Outport  Port=2
  FROC : Outport  Port=3
  wires:
  Mux5/1 -> Phasors/1
  Demux7/4 -> [Phase_Va]
  Demux7/1 -> [Mag_Va]
  Demux7/2 -> [Mag_Vb]
  Demux7/3 -> [Mag_Vc]
  Subsystem/1(Phasors_Vabc) -> Demux7/1
  Demux7/6 -> [Phase_Vc]
  Demux7/5 -> [Phase_Vb]
  Subsystem/3(Phasor_Freq) -> Phasor_Freq/1
  Measurements/1 -> Subsystem/1(Measurements1)
  Subsystem/4(Phasor_DTFreq) -> FROC/1
  Demux8/2 -> [Mag_Ib]
  Demux8/4 -> [Phase_Ia]
  Demux8/5 -> [Phase_Ib]
  Subsystem/2(Phasors_Iabc) -> Demux8/1
  Demux8/3 -> [Mag_Ic]
  Demux8/1 -> [Mag_Ia]
  Demux8/6 -> [Phase_Ic]
  [Phase_Ic] -> Mux5/12
  [Mag_Ic] -> Mux5/11
  [Phase_Ib] -> Mux5/10
  [Mag_Ib] -> Mux5/9
  [Phase_Ia] -> Mux5/8
  [Mag_Ia] -> Mux5/7
  [Phase_Vc] -> Mux5/6
  [Mag_Vc] -> Mux5/5
  [Phase_Vb] -> Mux5/4
  [Mag_Vb] -> Mux5/3
  [Phase_Va] -> Mux5/2
  [Mag_Va] -> Mux5/1

== system Feeder_1/SS_PMU/Subsystem19 ==
  Measurements : Inport
  Demux7 : Demux  Outputs=6
  Demux8 : Demux  Outputs=6
  Mux5 : Mux  Inputs=12
  Subsystem : Subsystem
  Phasors : Outport
  Phasor_Freq : Outport  Port=2
  FROC : Outport  Port=3
  wires:
  Mux5/1 -> Phasors/1
  Demux7/4 -> [Phase_Va]
  Demux7/1 -> [Mag_Va]
  Demux7/2 -> [Mag_Vb]
  Demux7/3 -> [Mag_Vc]
  Subsystem/1(Phasors_Vabc) -> Demux7/1
  Demux7/6 -> [Phase_Vc]
  Demux7/5 -> [Phase_Vb]
  Subsystem/3(Phasor_Freq) -> Phasor_Freq/1
  Measurements/1 -> Subsystem/1(Measurements1)
  Subsystem/4(Phasor_DTFreq) -> FROC/1
  Demux8/2 -> [Mag_Ib]
  Demux8/4 -> [Phase_Ia]
  Demux8/5 -> [Phase_Ib]
  Subsystem/2(Phasors_Iabc) -> Demux8/1
  Demux8/3 -> [Mag_Ic]
  Demux8/1 -> [Mag_Ia]
  Demux8/6 -> [Phase_Ic]
  [Phase_Ic] -> Mux5/12
  [Mag_Ic] -> Mux5/11
  [Phase_Ib] -> Mux5/10
  [Mag_Ib] -> Mux5/9
  [Phase_Ia] -> Mux5/8
  [Mag_Ia] -> Mux5/7
  [Phase_Vc] -> Mux5/6
  [Mag_Vc] -> Mux5/5
  [Phase_Vb] -> Mux5/4
  [Mag_Vb] -> Mux5/3
  [Phase_Va] -> Mux5/2
  [Mag_Va] -> Mux5/1

== system Feeder_1/SS_PMU/Subsystem2 ==
  Measurements : Inport
  Demux7 : Demux  Outputs=6
  Demux8 : Demux  Outputs=6
  Mux5 : Mux  Inputs=12
  Subsystem : Subsystem
  Phasors : Outport
  Phasor_Freq : Outport  Port=2
  FROC : Outport  Port=3
  wires:
  Mux5/1 -> Phasors/1
  Demux7/4 -> [Phase_Va]
  Demux7/1 -> [Mag_Va]
  Demux7/2 -> [Mag_Vb]
  Demux7/3 -> [Mag_Vc]
  Subsystem/1(Phasors_Vabc) -> Demux7/1
  Demux7/6 -> [Phase_Vc]
  Demux7/5 -> [Phase_Vb]
  Subsystem/3(Phasor_Freq) -> Phasor_Freq/1
  Measurements/1 -> Subsystem/1(Measurements1)
  Subsystem/4(Phasor_DTFreq) -> FROC/1
  Demux8/2 -> [Mag_Ib]
  Demux8/4 -> [Phase_Ia]
  Demux8/5 -> [Phase_Ib]
  Subsystem/2(Phasors_Iabc) -> Demux8/1
  Demux8/3 -> [Mag_Ic]
  Demux8/1 -> [Mag_Ia]
  Demux8/6 -> [Phase_Ic]
  [Phase_Ic] -> Mux5/12
  [Mag_Ic] -> Mux5/11
  [Phase_Ib] -> Mux5/10
  [Mag_Ib] -> Mux5/9
  [Phase_Ia] -> Mux5/8
  [Mag_Ia] -> Mux5/7
  [Phase_Vc] -> Mux5/6
  [Mag_Vc] -> Mux5/5
  [Phase_Vb] -> Mux5/4
  [Mag_Vb] -> Mux5/3
  [Phase_Va] -> Mux5/2
  [Mag_Va] -> Mux5/1

== system Feeder_1/SS_PMU/Subsystem20 ==
  Measurements : Inport
  Demux7 : Demux  Outputs=6
  Demux8 : Demux  Outputs=6
  Mux5 : Mux  Inputs=12
  Subsystem : Subsystem
  Phasors : Outport
  Phasor_Freq : Outport  Port=2
  FROC : Outport  Port=3
  wires:
  Mux5/1 -> Phasors/1
  Demux7/4 -> [Phase_Va]
  Demux7/1 -> [Mag_Va]
  Demux7/2 -> [Mag_Vb]
  Demux7/3 -> [Mag_Vc]
  Subsystem/1(Phasors_Vabc) -> Demux7/1
  Demux7/6 -> [Phase_Vc]
  Demux7/5 -> [Phase_Vb]
  Subsystem/3(Phasor_Freq) -> Phasor_Freq/1
  Measurements/1 -> Subsystem/1(Measurements1)
  Subsystem/4(Phasor_DTFreq) -> FROC/1
  Demux8/2 -> [Mag_Ib]
  Demux8/4 -> [Phase_Ia]
  Demux8/5 -> [Phase_Ib]
  Subsystem/2(Phasors_Iabc) -> Demux8/1
  Demux8/3 -> [Mag_Ic]
  Demux8/1 -> [Mag_Ia]
  Demux8/6 -> [Phase_Ic]
  [Phase_Ic] -> Mux5/12
  [Mag_Ic] -> Mux5/11
  [Phase_Ib] -> Mux5/10
  [Mag_Ib] -> Mux5/9
  [Phase_Ia] -> Mux5/8
  [Mag_Ia] -> Mux5/7
  [Phase_Vc] -> Mux5/6
  [Mag_Vc] -> Mux5/5
  [Phase_Vb] -> Mux5/4
  [Mag_Vb] -> Mux5/3
  [Phase_Va] -> Mux5/2
  [Mag_Va] -> Mux5/1

== system Feeder_1/SS_PMU/Subsystem21 ==
  Measurements : Inport
  Demux7 : Demux  Outputs=6
  Demux8 : Demux  Outputs=6
  Mux5 : Mux  Inputs=12
  Subsystem : Subsystem
  Phasors : Outport
  Phasor_Freq : Outport  Port=2
  FROC : Outport  Port=3
  wires:
  Mux5/1 -> Phasors/1
  Demux7/4 -> [Phase_Va]
  Demux7/1 -> [Mag_Va]
  Demux7/2 -> [Mag_Vb]
  Demux7/3 -> [Mag_Vc]
  Subsystem/1(Phasors_Vabc) -> Demux7/1
  Demux7/6 -> [Phase_Vc]
  Demux7/5 -> [Phase_Vb]
  Subsystem/3(Phasor_Freq) -> Phasor_Freq/1
  Measurements/1 -> Subsystem/1(Measurements1)
  Subsystem/4(Phasor_DTFreq) -> FROC/1
  Demux8/2 -> [Mag_Ib]
  Demux8/4 -> [Phase_Ia]
  Demux8/5 -> [Phase_Ib]
  Subsystem/2(Phasors_Iabc) -> Demux8/1
  Demux8/3 -> [Mag_Ic]
  Demux8/1 -> [Mag_Ia]
  Demux8/6 -> [Phase_Ic]
  [Phase_Ic] -> Mux5/12
  [Mag_Ic] -> Mux5/11
  [Phase_Ib] -> Mux5/10
  [Mag_Ib] -> Mux5/9
  [Phase_Ia] -> Mux5/8
  [Mag_Ia] -> Mux5/7
  [Phase_Vc] -> Mux5/6
  [Mag_Vc] -> Mux5/5
  [Phase_Vb] -> Mux5/4
  [Mag_Vb] -> Mux5/3
  [Phase_Va] -> Mux5/2
  [Mag_Va] -> Mux5/1

== system Feeder_1/SS_PMU/Subsystem22 ==
  Measurements : Inport
  Demux7 : Demux  Outputs=6
  Demux8 : Demux  Outputs=6
  Mux5 : Mux  Inputs=12
  Subsystem : Subsystem
  Phasors : Outport
  Phasor_Freq : Outport  Port=2
  FROC : Outport  Port=3
  wires:
  Mux5/1 -> Phasors/1
  Demux7/4 -> [Phase_Va]
  Demux7/1 -> [Mag_Va]
  Demux7/2 -> [Mag_Vb]
  Demux7/3 -> [Mag_Vc]
  Subsystem/1(Phasors_Vabc) -> Demux7/1
  Demux7/6 -> [Phase_Vc]
  Demux7/5 -> [Phase_Vb]
  Subsystem/3(Phasor_Freq) -> Phasor_Freq/1
  Measurements/1 -> Subsystem/1(Measurements1)
  Subsystem/4(Phasor_DTFreq) -> FROC/1
  Demux8/2 -> [Mag_Ib]
  Demux8/4 -> [Phase_Ia]
  Demux8/5 -> [Phase_Ib]
  Subsystem/2(Phasors_Iabc) -> Demux8/1
  Demux8/3 -> [Mag_Ic]
  Demux8/1 -> [Mag_Ia]
  Demux8/6 -> [Phase_Ic]
  [Phase_Ic] -> Mux5/12
  [Mag_Ic] -> Mux5/11
  [Phase_Ib] -> Mux5/10
  [Mag_Ib] -> Mux5/9
  [Phase_Ia] -> Mux5/8
  [Mag_Ia] -> Mux5/7
  [Phase_Vc] -> Mux5/6
  [Mag_Vc] -> Mux5/5
  [Phase_Vb] -> Mux5/4
  [Mag_Vb] -> Mux5/3
  [Phase_Va] -> Mux5/2
  [Mag_Va] -> Mux5/1

== system Feeder_1/SS_PMU/Subsystem23 ==
  PMU in : Inport
  Bus Selector : BusSelector  OutputSignals=Measurements,FREQ,FROC
  Constant28 : Constant  Value=-1
  Constant29 : Constant  Value=-1
  Subsystem : Subsystem
  Phasors : Outport
  Analog : Outport  Port=2
  Ditigal : Outport  Port=3
  FREQ : Outport  Port=4
  FROC : Outport  Port=5
  wires:
  Subsystem/1(Out1) -> Bus Selector/1
  Bus Selector/1 -> Phasors/1  "<Measurements>"
  PMU in/1 -> Subsystem/1(In1)
  Constant28/1 -> Analog/1
  Constant29/1 -> Ditigal/1
  Bus Selector/2 -> FREQ/1  "<FREQ>"
  Bus Selector/3 -> FROC/1  "<FROC>"

== system Feeder_1/SS_PMU/Subsystem24 ==
  PMU in : Inport
  Bus Selector : BusSelector  OutputSignals=Measurements,FREQ,FROC
  Constant28 : Constant  Value=-1
  Constant29 : Constant  Value=-1
  Subsystem : Subsystem
  Phasors : Outport
  Analog : Outport  Port=2
  Ditigal : Outport  Port=3
  FREQ : Outport  Port=4
  FROC : Outport  Port=5
  wires:
  Subsystem/1(Out1) -> Bus Selector/1
  Bus Selector/1 -> Phasors/1  "<Measurements>"
  PMU in/1 -> Subsystem/1(In1)
  Constant28/1 -> Analog/1
  Constant29/1 -> Ditigal/1
  Bus Selector/2 -> FREQ/1  "<FREQ>"
  Bus Selector/3 -> FROC/1  "<FROC>"

== system Feeder_1/SS_PMU/Subsystem25 ==
  PMU in : Inport
  Bus Selector : BusSelector  OutputSignals=Measurements,FREQ,FROC
  Constant28 : Constant  Value=-1
  Constant29 : Constant  Value=-1
  Subsystem : Subsystem
  Phasors : Outport
  Analog : Outport  Port=2
  Ditigal : Outport  Port=3
  FREQ : Outport  Port=4
  FROC : Outport  Port=5
  wires:
  Subsystem/1(Out1) -> Bus Selector/1
  Bus Selector/1 -> Phasors/1  "<Measurements>"
  PMU in/1 -> Subsystem/1(In1)
  Constant28/1 -> Analog/1
  Constant29/1 -> Ditigal/1
  Bus Selector/2 -> FREQ/1  "<FREQ>"
  Bus Selector/3 -> FROC/1  "<FROC>"

== system Feeder_1/SS_PMU/Subsystem26 ==
  PMU in : Inport
  Bus Selector : BusSelector  OutputSignals=Measurements,FREQ,FROC
  Constant28 : Constant  Value=-1
  Constant29 : Constant  Value=-1
  Subsystem : Subsystem
  Phasors : Outport
  Analog : Outport  Port=2
  Ditigal : Outport  Port=3
  FREQ : Outport  Port=4
  FROC : Outport  Port=5
  wires:
  Subsystem/1(Out1) -> Bus Selector/1
  Bus Selector/1 -> Phasors/1  "<Measurements>"
  PMU in/1 -> Subsystem/1(In1)
  Constant28/1 -> Analog/1
  Constant29/1 -> Ditigal/1
  Bus Selector/2 -> FREQ/1  "<FREQ>"
  Bus Selector/3 -> FROC/1  "<FROC>"

== system Feeder_1/SS_PMU/Subsystem27 ==
  PMU in : Inport
  Bus Selector : BusSelector  OutputSignals=Measurements,FREQ,FROC
  Constant28 : Constant  Value=-1
  Constant29 : Constant  Value=-1
  Subsystem : Subsystem
  Phasors : Outport
  Analog : Outport  Port=2
  Ditigal : Outport  Port=3
  FREQ : Outport  Port=4
  FROC : Outport  Port=5
  wires:
  Subsystem/1(Out1) -> Bus Selector/1
  Bus Selector/1 -> Phasors/1  "<Measurements>"
  PMU in/1 -> Subsystem/1(In1)
  Constant28/1 -> Analog/1
  Constant29/1 -> Ditigal/1
  Bus Selector/2 -> FREQ/1  "<FREQ>"
  Bus Selector/3 -> FROC/1  "<FROC>"

== system Feeder_1/SS_PMU/Subsystem28 ==
  PMU in : Inport
  Bus Selector : BusSelector  OutputSignals=Measurements,FREQ,FROC
  Constant28 : Constant  Value=-1
  Constant29 : Constant  Value=-1
  Subsystem : Subsystem
  Phasors : Outport
  Analog : Outport  Port=2
  Ditigal : Outport  Port=3
  FREQ : Outport  Port=4
  FROC : Outport  Port=5
  wires:
  Subsystem/1(Out1) -> Bus Selector/1
  Bus Selector/1 -> Phasors/1  "<Measurements>"
  PMU in/1 -> Subsystem/1(In1)
  Constant28/1 -> Analog/1
  Constant29/1 -> Ditigal/1
  Bus Selector/2 -> FREQ/1  "<FREQ>"
  Bus Selector/3 -> FROC/1  "<FROC>"

== system Feeder_1/SS_PMU/Subsystem29 ==
  PMU in : Inport
  Bus Selector : BusSelector  OutputSignals=Measurements,FREQ,FROC
  Constant28 : Constant  Value=-1
  Constant29 : Constant  Value=-1
  Subsystem : Subsystem
  Phasors : Outport
  Analog : Outport  Port=2
  Ditigal : Outport  Port=3
  FREQ : Outport  Port=4
  FROC : Outport  Port=5
  wires:
  Subsystem/1(Out1) -> Bus Selector/1
  Bus Selector/1 -> Phasors/1  "<Measurements>"
  PMU in/1 -> Subsystem/1(In1)
  Constant28/1 -> Analog/1
  Constant29/1 -> Ditigal/1
  Bus Selector/2 -> FREQ/1  "<FREQ>"
  Bus Selector/3 -> FROC/1  "<FROC>"

== system Feeder_1/SS_PMU/Subsystem3 ==
  Measurements : Inport
  Demux7 : Demux  Outputs=6
  Demux8 : Demux  Outputs=6
  Mux5 : Mux  Inputs=12
  Subsystem : Subsystem
  Phasors : Outport
  Phasor_Freq : Outport  Port=2
  FROC : Outport  Port=3
  wires:
  Mux5/1 -> Phasors/1
  Demux7/4 -> [Phase_Va]
  Demux7/1 -> [Mag_Va]
  Demux7/2 -> [Mag_Vb]
  Demux7/3 -> [Mag_Vc]
  Subsystem/1(Phasors_Vabc) -> Demux7/1
  Demux7/6 -> [Phase_Vc]
  Demux7/5 -> [Phase_Vb]
  Subsystem/3(Phasor_Freq) -> Phasor_Freq/1
  Measurements/1 -> Subsystem/1(Measurements1)
  Subsystem/4(Phasor_DTFreq) -> FROC/1
  Demux8/2 -> [Mag_Ib]
  Demux8/4 -> [Phase_Ia]
  Demux8/5 -> [Phase_Ib]
  Subsystem/2(Phasors_Iabc) -> Demux8/1
  Demux8/3 -> [Mag_Ic]
  Demux8/1 -> [Mag_Ia]
  Demux8/6 -> [Phase_Ic]
  [Phase_Ic] -> Mux5/12
  [Mag_Ic] -> Mux5/11
  [Phase_Ib] -> Mux5/10
  [Mag_Ib] -> Mux5/9
  [Phase_Ia] -> Mux5/8
  [Mag_Ia] -> Mux5/7
  [Phase_Vc] -> Mux5/6
  [Mag_Vc] -> Mux5/5
  [Phase_Vb] -> Mux5/4
  [Mag_Vb] -> Mux5/3
  [Phase_Va] -> Mux5/2
  [Mag_Va] -> Mux5/1

== system Feeder_1/SS_PMU/Subsystem30 ==
  PMU in : Inport
  Bus Selector : BusSelector  OutputSignals=Measurements,FREQ,FROC
  Constant28 : Constant  Value=-1
  Constant29 : Constant  Value=-1
  Subsystem : Subsystem
  Phasors : Outport
  Analog : Outport  Port=2
  Ditigal : Outport  Port=3
  FREQ : Outport  Port=4
  FROC : Outport  Port=5
  wires:
  Subsystem/1(Out1) -> Bus Selector/1
  Bus Selector/1 -> Phasors/1  "<Measurements>"
  PMU in/1 -> Subsystem/1(In1)
  Constant28/1 -> Analog/1
  Constant29/1 -> Ditigal/1
  Bus Selector/2 -> FREQ/1  "<FREQ>"
  Bus Selector/3 -> FROC/1  "<FROC>"

== system Feeder_1/SS_PMU/Subsystem31 ==
  PMU in : Inport
  Bus Selector : BusSelector  OutputSignals=Measurements,FREQ,FROC
  Constant28 : Constant  Value=-1
  Constant29 : Constant  Value=-1
  Subsystem : Subsystem
  Phasors : Outport
  Analog : Outport  Port=2
  Ditigal : Outport  Port=3
  FREQ : Outport  Port=4
  FROC : Outport  Port=5
  wires:
  Subsystem/1(Out1) -> Bus Selector/1
  Bus Selector/1 -> Phasors/1  "<Measurements>"
  PMU in/1 -> Subsystem/1(In1)
  Constant28/1 -> Analog/1
  Constant29/1 -> Ditigal/1
  Bus Selector/2 -> FREQ/1  "<FREQ>"
  Bus Selector/3 -> FROC/1  "<FROC>"

== system Feeder_1/SS_PMU/Subsystem32 ==
  PMU in : Inport
  Bus Selector : BusSelector  OutputSignals=Measurements,FREQ,FROC
  Constant28 : Constant  Value=-1
  Constant29 : Constant  Value=-1
  Subsystem : Subsystem
  Phasors : Outport
  Analog : Outport  Port=2
  Ditigal : Outport  Port=3
  FREQ : Outport  Port=4
  FROC : Outport  Port=5
  wires:
  Subsystem/1(Out1) -> Bus Selector/1
  Bus Selector/1 -> Phasors/1  "<Measurements>"
  PMU in/1 -> Subsystem/1(In1)
  Constant28/1 -> Analog/1
  Constant29/1 -> Ditigal/1
  Bus Selector/2 -> FREQ/1  "<FREQ>"
  Bus Selector/3 -> FROC/1  "<FROC>"

== system Feeder_1/SS_PMU/Subsystem33 ==
  PMU in : Inport
  Bus Selector : BusSelector  OutputSignals=Measurements,FREQ,FROC
  Constant28 : Constant  Value=-1
  Constant29 : Constant  Value=-1
  Subsystem : Subsystem
  Phasors : Outport
  Analog : Outport  Port=2
  Ditigal : Outport  Port=3
  FREQ : Outport  Port=4
  FROC : Outport  Port=5
  wires:
  Subsystem/1(Out1) -> Bus Selector/1
  Bus Selector/1 -> Phasors/1  "<Measurements>"
  PMU in/1 -> Subsystem/1(In1)
  Constant28/1 -> Analog/1
  Constant29/1 -> Ditigal/1
  Bus Selector/2 -> FREQ/1  "<FREQ>"
  Bus Selector/3 -> FROC/1  "<FROC>"

== system Feeder_1/SS_PMU/Subsystem34 ==
  PMU in : Inport
  Bus Selector : BusSelector  OutputSignals=Measurements,FREQ,FROC
  Constant28 : Constant  Value=-1
  Constant29 : Constant  Value=-1
  Subsystem : Subsystem
  Phasors : Outport
  Analog : Outport  Port=2
  Ditigal : Outport  Port=3
  FREQ : Outport  Port=4
  FROC : Outport  Port=5
  wires:
  Subsystem/1(Out1) -> Bus Selector/1
  Bus Selector/1 -> Phasors/1  "<Measurements>"
  PMU in/1 -> Subsystem/1(In1)
  Constant28/1 -> Analog/1
  Constant29/1 -> Ditigal/1
  Bus Selector/2 -> FREQ/1  "<FREQ>"
  Bus Selector/3 -> FROC/1  "<FROC>"
